simulink model "SpeedandDirection"  (R2022a)
settings: Solver=VariableStepAuto  StartTime=0.0  StopTime=10.0  RelTol=1e-3
libraries: arduinolib x2
settings Model: Creator=sokse  LastModifiedBy=sokse

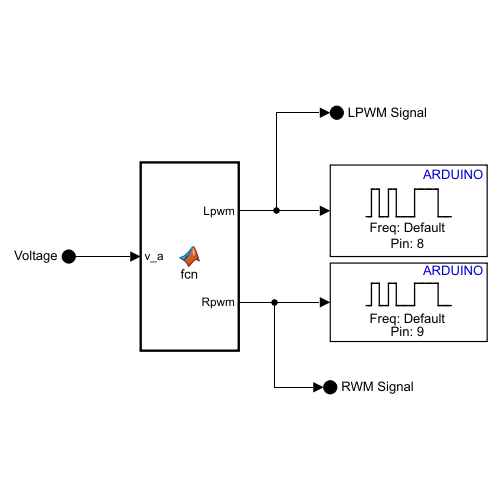
[thumbnail: Simulink's stored preview of the top-level diagram]
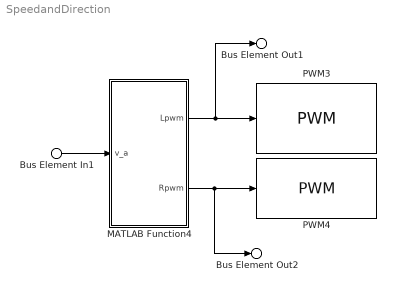
== system SpeedandDirection ==
  Bus Element In1 : Inport  PortName=Voltage
  MATLAB Function4 : MATLAB Function  TreatAsAtomicUnit=on
  PWM3 : arduinolib/PWM  pinNumber=8  frequencyType=Default  desiredFrequency=490.2  achievableFrequency=490.2
  PWM4 : arduinolib/PWM  pinNumber=9  frequencyType=Default  desiredFrequency=490.2  achievableFrequency=490.2
  Bus Element Out1 : Outport  PortName=LPWM Signal
  Bus Element Out2 : Outport  Port=2  PortName=RPWM Signal
  wires:
  Bus Element In1/1 -> MATLAB Function4/1(v_a)
  MATLAB Function4/1(Lpwm) -> Bus Element Out1/1, PWM3/1
  MATLAB Function4/2(Rpwm) -> Bus Element Out2/1, PWM4/1

== matlab function SpeedandDirection/MATLAB Function4 ==
  data: v_a input; Lpwm output; Rpwm output
function [Lpwm,Rpwm] = fcn(v_a)

vmax = 22.9;
pwm_cal = v_a*254/vmax;

if pwm_cal > 0
    Lpwm = 0;
    Rpwm = pwm_cal;
elseif pwm_cal < 0
    Lpwm = abs(pwm_cal);
    Rpwm = 0;
else
    Lpwm = 0;
    Rpwm = 0;
end
